simulink model "chap11_1sim"  (Simulink 6.3)
settings: Solver=ode45  StartTime=0.0  StopTime=20  RelTol=1e-3
settings Model: LastModifiedBy=Administrator  ExtModeTrigMode=oneshot  ExtModeArmWhenConnect=off  StrictBusMsg=None
settings DataIOCC: LimitDataPoints=off
settings OptimizationCC: BlockReduction=off  BooleanDataType=off
settings DebuggingCC: SolverPrmCheckMsg=none
settings HardwareCC: TargetUnknown=on

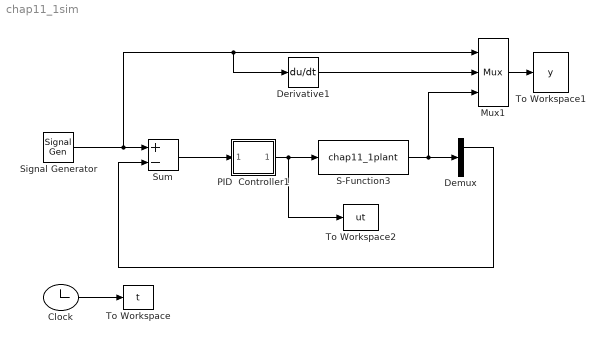
== system chap11_1sim ==
  Clock : Clock
  Demux : Demux  Outputs=2
  Derivative1 : Derivative
  Mux1 : Mux  Inputs=3
  PID  Controller1 : Subsystem  mask(PID Controller){@1=20, @2=0, @3=5}
      mask prompts: @1 "Proportional:"; @2 "Integral"; @3 "Derivative:"
      mask help:
      | Enter expressions for proportional, integral, and derivative terms.
      | P+I/s+Ds
      mask init:
      | P=@1; I=@2; D=@3;
      mask Help: This block implements a PID controller where parameters are entered for the Proportional, Integral and Derivative terms. Unmask this block to see how it works. The derivative term is implemented using a true derivative block.
      mask Display: disp('PID')
  S-Function3 : S-Function  FunctionName=chap11_1plant
  Signal Generator : SignalGenerator  Amplitude=0.1  Frequency=0.10
  Sum : Sum  Inputs=+-  SaturateOnIntegerOverflow=on  InputSameDT=on
  To Workspace : ToWorkspace  VariableName=t  SampleTime=-1  SaveFormat=Array
  To Workspace1 : ToWorkspace  VariableName=y  SampleTime=-1  SaveFormat=Array
  To Workspace2 : ToWorkspace  VariableName=ut  SampleTime=-1  SaveFormat=Array
  wires:
  Sum/1 -> PID  Controller1/1(In_1)
  Signal Generator/1 -> Sum/1, Derivative1/1, Mux1/1
  Mux1/1 -> To Workspace1/1
  PID  Controller1/1(Out_1) -> S-Function3/1, To Workspace2/1
  Clock/1 -> To Workspace/1
  Derivative1/1 -> Mux1/2
  S-Function3/1 -> Demux/1, Mux1/3
  Demux/1 -> Sum/2

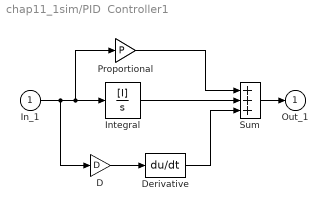
== system chap11_1sim/PID  Controller1 ==
  In_1 : Inport
  D : Gain  Gain=D  SaturateOnIntegerOverflow=on
  Derivative : Derivative
  Integral : TransferFcn  Numerator=[I]  Denominator=[1 0]
  Proportional : Gain  Gain=P  SaturateOnIntegerOverflow=on
  Sum : Sum  Inputs=+++  SaturateOnIntegerOverflow=on  InputSameDT=on
  Out_1 : Outport  InitialOutput=0
  wires:
  D/1 -> Derivative/1
  Sum/1 -> Out_1/1
  In_1/1 -> D/1, Proportional/1, Integral/1
  Derivative/1 -> Sum/3
  Integral/1 -> Sum/2
  Proportional/1 -> Sum/1
